simulink model "PracticaPotencia"  (R2024b)
settings: Solver=VariableStepAuto  StartTime=0.0  StopTime=200e-3  MaxStep=1e-4  RelTol=1e-3
libraries: spsVoltageMeasurementLib x14, spsDiodeLib x12, spsCurrentMeasurementLib x8, spsParallelRLCBranchLib x5, spsThreePhaseProgrammableVoltageSourceLib x2, spsMeanLib x1, spsRMSLib x1, sps_lib x1, spspowerguiLib x1
settings Model: Creator=javier  LastModifiedBy=javier

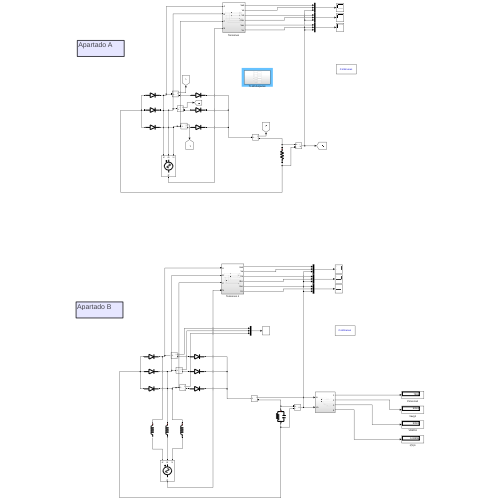
[thumbnail: Simulink's stored preview of the top-level diagram]
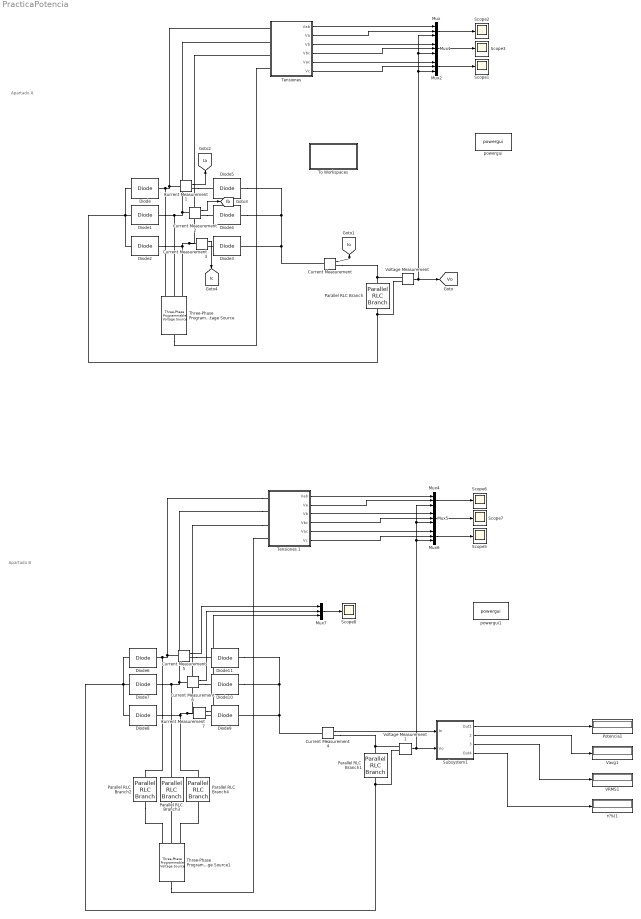
== system PracticaPotencia ==
  note: Apartado A
  note: Apartado B
  Current Measurement{,1..7} (8 alike) : spsCurrentMeasurementLib/Current Measurement  PhasorSimulation=off  OutputType=Complex  PSBequivalent=0
  Diode{,1..11} (12 alike) : spsDiodeLib/Diode  Ron=0.001  Lon=0  Vf=0.8  IC=0  UseSnubber=0  Rs=500  Cs=250e-9  Measurements=off
  Mux{,1..2,4..7} (7 alike) : Mux  Inputs=3
  Parallel RLC Branch : spsParallelRLCBranchLib/Parallel RLC Branch  LConnTagsString=a  RConnTagsString=__new0  BranchType=R  Resistance=30  Inductance=1e-3  SetiL0=off  InitialCurrent=0  Capacitance=1e-6  Setx0=off  InitialVoltage=0  Measurements=None
  Parallel RLC Branch1 : spsParallelRLCBranchLib/Parallel RLC Branch  LConnTagsString=a  RConnTagsString=__new0  BranchType=RC  Resistance=30  Inductance=1e-3  SetiL0=off  InitialCurrent=0  Capacitance=10e-3  Setx0=off  InitialVoltage=0  Measurements=None
  Parallel RLC Branch2 : spsParallelRLCBranchLib/Parallel RLC Branch  LConnTagsString=a  RConnTagsString=__new0  BranchType=L  Resistance=30  Inductance=5e-3  SetiL0=off  InitialCurrent=0  Capacitance=1e-6  Setx0=off  InitialVoltage=0  Measurements=None
  Parallel RLC Branch3 : spsParallelRLCBranchLib/Parallel RLC Branch  LConnTagsString=a  RConnTagsString=__new0  BranchType=L  Resistance=30  Inductance=5e-3  SetiL0=off  InitialCurrent=0  Capacitance=1e-6  Setx0=off  InitialVoltage=0  Measurements=None
  Parallel RLC Branch4 : spsParallelRLCBranchLib/Parallel RLC Branch  LConnTagsString=a  RConnTagsString=__new0  BranchType=L  Resistance=30  Inductance=5e-3  SetiL0=off  InitialCurrent=0  Capacitance=1e-6  Setx0=off  InitialVoltage=0  Measurements=None
  Potencia1 : Display
  Scope{1..3,5..8} (7 alike) : Scope
  Subsystem1 : Subsystem
  "Tensiones " : Subsystem
  Tensiones 1 : Subsystem
  Three-Phase Programmable Voltage Source : spsThreePhaseProgrammableVoltageSourceLib/Three-Phase Programmable Voltage Source  PositiveSequence="[400  0 50]"  VariationEntity=None  VariationType=Table of time-amplitude pairs  VariationTypeAlt=Step  VariationStep=0.5  VariationRate=10  VariationMagnitude=0.3  VariationFrequency=2  VariationTiming=[1 2]  VariationPhaseA=off  Amplitudes=[1 0.8 1.2 1.0]  TimeValues=[0 0.1 0.15 0.2]  HarmonicGeneration=off  HarmonicA=[3 0.2 -25 0]  HarmonicB=[2 0.15 35 2]  Timing="[0.05  3]"  BusType=swing  Pref=0  Qref=0  Qmin=-inf  Qmax=inf
  Three-Phase Programmable Voltage Source1 : spsThreePhaseProgrammableVoltageSourceLib/Three-Phase Programmable Voltage Source  PositiveSequence="[400  0 50]"  VariationEntity=None  VariationType=Table of time-amplitude pairs  VariationTypeAlt=Step  VariationStep=0.5  VariationRate=10  VariationMagnitude=0.3  VariationFrequency=2  VariationTiming=[1 2]  VariationPhaseA=off  Amplitudes=[1 0.8 1.2 1.0]  TimeValues=[0 0.1 0.15 0.2]  HarmonicGeneration=off  HarmonicA=[3 0.2 -25 0]  HarmonicB=[2 0.15 35 2]  Timing="[0.05  3]"  BusType=swing  Pref=0  Qref=0  Qmin=-inf  Qmax=inf
  To Workspaces : Subsystem
  VRMS1 : Display
  Vavg1 : Display
  Voltage Measurement : spsVoltageMeasurementLib/Voltage Measurement  PhasorSimulation=off  OutputType=Complex  PSBequivalent=0
  Voltage Measurement1 : spsVoltageMeasurementLib/Voltage Measurement  PhasorSimulation=off  OutputType=Complex  PSBequivalent=0
  powergui : sps_lib/powergui  Priority=1  SimulationMode=Continuous  SampleTime=50e-6  frequency=60  Iterations=50  frequencyindice=50  Pbase=100e6  ErrMax=1e-4  UnitsV=kV  UnitsW=MW  buscounter=0  FunctionMessages=off  echomessages=off  EnableUseOfTLC=off  CurrentSourceSwitches=off  DisableSnubberDevices=on  DisableRonSwitches=off  DisableVfSwitches=off  DisplayEquations=off  AutomaticDiscreteSolvers=off  SolverType=Tustin/Backward Euler (TBE)  Interpol=off  ExternalGateDelay=off  methode=off  Ts=100  x0status=blocks  SPID=on  SwTol=0  HookPort=off  NonlinearTolerance=1e-4  nMaxIteration=100  ContinueOnMaxIteration=off  RestoreLinks=warning  ResistiveCurrentMeasurement=off  Frange=[0:2:500]  Ylog=off  Xlog=on  ShowGrid=off  save=off  variable=ZData  structure=0  ZoomFFT=off  StartTime=0.0  cycles=1  DisplayStyle=1  fundamental=60  FreqAxis=off  MaxFrequency=1000  frequencyindicesteady=1  RmsSteady=1  display=off
  powergui1 : spspowerguiLib/powergui  Priority=1  SimulationMode=Continuous  SampleTime=50e-6  frequency=60  Iterations=50  frequencyindice=50  Pbase=100e6  ErrMax=1e-4  UnitsV=kV  UnitsW=MW  buscounter=0  FunctionMessages=off  echomessages=off  EnableUseOfTLC=off  CurrentSourceSwitches=off  DisableSnubberDevices=on  DisableRonSwitches=off  DisableVfSwitches=off  DisplayEquations=off  AutomaticDiscreteSolvers=off  SolverType=Tustin/Backward Euler (TBE)  Interpol=off  ExternalGateDelay=off  methode=off  Ts=100  x0status=blocks  SPID=on  SwTol=0  HookPort=off  NonlinearTolerance=1e-4  nMaxIteration=100  ContinueOnMaxIteration=off  RestoreLinks=warning  ResistiveCurrentMeasurement=off  Frange=[0:2:500]  Ylog=off  Xlog=on  ShowGrid=off  save=off  variable=ZData  structure=0  ZoomFFT=off  StartTime=0.0  cycles=1  DisplayStyle=1  fundamental=60  FreqAxis=off  MaxFrequency=1000  frequencyindicesteady=1  RmsSteady=1  display=off
  r(%)1 : Display
  tag scope: Ia=global, Ib=global, Ic=global, Io=global, Vo=global
  wires:
  Voltage Measurement/1 -> [Vo], Mux1/3, Mux/3, Mux2/3
  "Tensiones "/1(Vab) -> Mux/1
  "Tensiones "/2(Va) -> Mux/2
  "Tensiones "/3(Vb) -> Mux1/1
  "Tensiones "/4(Vbc) -> Mux1/2
  "Tensiones "/5(Vac) -> Mux2/1
  "Tensiones "/6(Vc) -> Mux2/2
  Mux/1 -> Scope2/1
  Mux1/1 -> Scope3/1
  Mux2/1 -> Scope1/1
  Current Measurement1/1 -> [Ia]
  Tensiones 1/1(Vab) -> Mux4/1
  Tensiones 1/6(Vc) -> Mux6/2
  Current Measurement4/1 -> Subsystem1/1(Io)
  Tensiones 1/3(Vb) -> Mux5/1
  Mux7/1 -> Scope8/1
  Tensiones 1/5(Vac) -> Mux6/1
  Current Measurement5/1 -> Mux7/1
  Subsystem1/2(2) -> Vavg1/1
  Mux5/1 -> Scope7/1
  Voltage Measurement1/1 -> Subsystem1/2(Vo), Mux5/3, Mux4/3, Mux6/3
  Mux6/1 -> Scope5/1
  Subsystem1/1(Out1) -> Potencia1/1
  Subsystem1/4(Out4) -> r(%)1/1
  Subsystem1/3(3) -> VRMS1/1
  Mux4/1 -> Scope6/1
  Current Measurement6/1 -> Mux7/2
  Current Measurement7/1 -> Mux7/3
  Tensiones 1/4(Vbc) -> Mux5/2
  Tensiones 1/2(Va) -> Mux4/2
  Current Measurement/1 -> [Io]
  Current Measurement2/1 -> [Ib]
  Current Measurement3/1 -> [Ic]
  connections:
  Voltage Measurement/LConn2 -- Parallel RLC Branch/RConn1 -- Diode2/LConn1 -- Diode1/LConn1 -- Diode/LConn1
  Diode5/RConn1 -- Current Measurement/LConn1 -- Diode3/RConn1 -- Diode4/RConn1
  Current Measurement/RConn1 -- Voltage Measurement/LConn1 -- Parallel RLC Branch/LConn1
  Three-Phase Programmable Voltage Source/LConn1 -- "Tensiones "/LConn4
  Diode/RConn1 -- Current Measurement1/LConn1 -- "Tensiones "/LConn1 -- Three-Phase Programmable Voltage Source/RConn1
  Diode1/RConn1 -- Current Measurement2/LConn1 -- "Tensiones "/LConn2 -- Three-Phase Programmable Voltage Source/RConn2
  Diode2/RConn1 -- Current Measurement3/LConn1 -- "Tensiones "/LConn3 -- Three-Phase Programmable Voltage Source/RConn3
  Current Measurement1/RConn1 -- Diode5/LConn1
  Current Measurement2/RConn1 -- Diode4/LConn1
  Current Measurement3/RConn1 -- Diode3/LConn1
  Tensiones 1/LConn1 -- Diode6/RConn1 -- Parallel RLC Branch2/LConn1 -- Current Measurement5/LConn1
  Tensiones 1/LConn2 -- Parallel RLC Branch3/LConn1 -- Diode7/RConn1 -- Current Measurement6/LConn1
  Diode6/LConn1 -- Voltage Measurement1/LConn2 -- Parallel RLC Branch1/RConn1 -- Diode8/LConn1 -- Diode7/LConn1
  Tensiones 1/LConn3 -- Parallel RLC Branch4/LConn1 -- Diode8/RConn1 -- Current Measurement7/LConn1
  Diode10/RConn1 -- Diode11/RConn1 -- Current Measurement4/LConn1 -- Diode9/RConn1
  Parallel RLC Branch1/LConn1 -- Current Measurement4/RConn1 -- Voltage Measurement1/LConn1
  Current Measurement6/RConn1 -- Diode10/LConn1
  Current Measurement7/RConn1 -- Diode9/LConn1
  Three-Phase Programmable Voltage Source1/LConn1 -- Tensiones 1/LConn4
  Current Measurement5/RConn1 -- Diode11/LConn1
  Parallel RLC Branch2/RConn1 -- Three-Phase Programmable Voltage Source1/RConn1
  Three-Phase Programmable Voltage Source1/RConn2 -- Parallel RLC Branch3/RConn1
  Three-Phase Programmable Voltage Source1/RConn3 -- Parallel RLC Branch4/RConn1

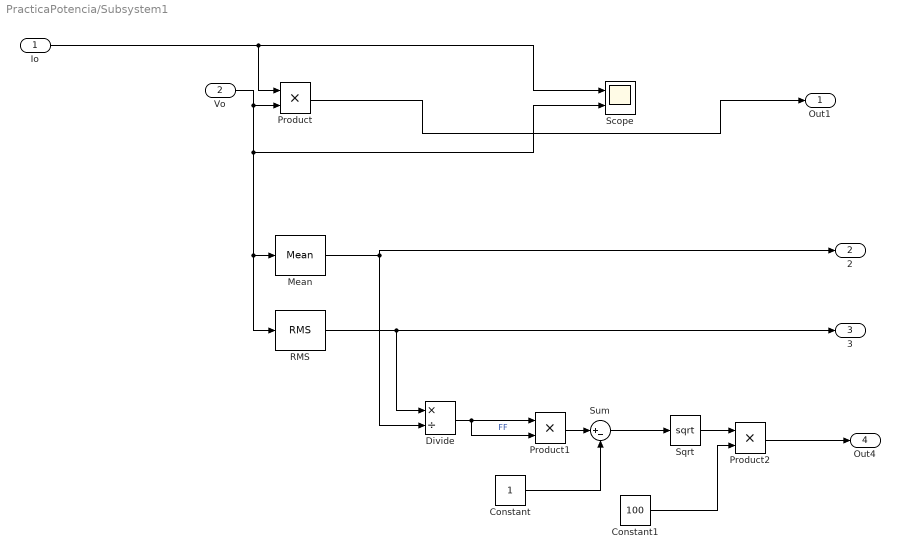
== system PracticaPotencia/Subsystem1 ==
  Io : Inport
  Vo : Inport  Port=2
  Constant : Constant
  Constant1 : Constant  Value=100
  Divide : Product  Inputs=*/
  Mean : spsMeanLib/Mean  Freq=50  Vinit=0  Ts=0
  Product : Product
  Product1 : Product
  Product2 : Product
  RMS : spsRMSLib/RMS  TrueRMS=on  Freq=50  RMSInit=120  Ts=0
  Scope : Scope  NumInputPorts=2
  Sqrt : Sqrt
  Sum : Sum  Inputs=|+-
  Out1 : Outport
  2 : Outport  Port=2
  3 : Outport  Port=3
  Out4 : Outport  Port=4
  wires:
  Vo/1 -> Scope/2, Mean/1, RMS/1, Product/2
  Constant/1 -> Sum/2
  Constant1/1 -> Product2/2
  RMS/1 -> 3/1, Divide/1
  Io/1 -> Scope/1, Product/1
  Divide/1 -> Product1/2, Product1/1  "FF"
  Sqrt/1 -> Product2/1
  Sum/1 -> Sqrt/1
  Mean/1 -> 2/1, Divide/2
  Product1/1 -> Sum/1
  Product/1 -> Out1/1
  Product2/1 -> Out4/1

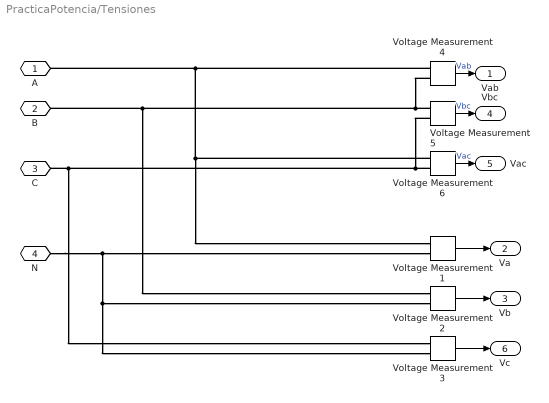
== system PracticaPotencia/Tensiones  ==
  Voltage Measurement{1..6} (6 alike) : spsVoltageMeasurementLib/Voltage Measurement  PhasorSimulation=off  OutputType=Complex  PSBequivalent=0
  A : PMIOPort  Side=Left
  B : PMIOPort  Port=2  Side=Left
  C : PMIOPort  Port=3  Side=Left
  N : PMIOPort  Port=4  Side=Left
  Vab : Outport
  Va : Outport  Port=2
  Vb : Outport  Port=3
  Vbc : Outport  Port=4
  Vac : Outport  Port=5
  Vc : Outport  Port=6
  wires:
  Voltage Measurement6/1 -> Vac/1  "Vac"
  Voltage Measurement5/1 -> Vbc/1  "Vbc"
  Voltage Measurement4/1 -> Vab/1  "Vab"
  Voltage Measurement1/1 -> Va/1
  Voltage Measurement2/1 -> Vb/1
  Voltage Measurement3/1 -> Vc/1
  connections:
  Voltage Measurement5/LConn2 -- Voltage Measurement6/LConn2 -- Voltage Measurement3/LConn1 -- C/RConn1
  Voltage Measurement4/LConn1 -- Voltage Measurement6/LConn1 -- Voltage Measurement1/LConn1 -- A/RConn1
  Voltage Measurement5/LConn1 -- Voltage Measurement4/LConn2 -- Voltage Measurement2/LConn1 -- B/RConn1
  N/RConn1 -- Voltage Measurement3/LConn2 -- Voltage Measurement2/LConn2 -- Voltage Measurement1/LConn2

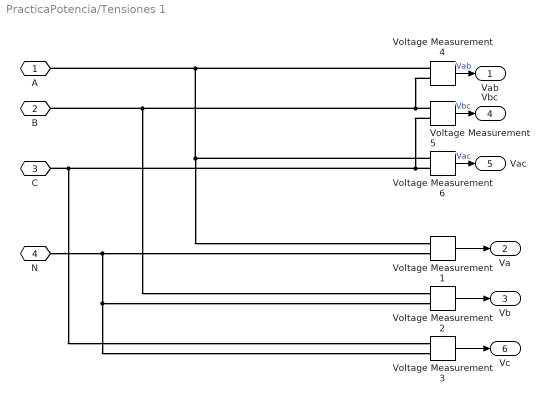
== system PracticaPotencia/Tensiones 1 ==
  Voltage Measurement{1..6} (6 alike) : spsVoltageMeasurementLib/Voltage Measurement  PhasorSimulation=off  OutputType=Complex  PSBequivalent=0
  A : PMIOPort  Side=Left
  B : PMIOPort  Port=2  Side=Left
  C : PMIOPort  Port=3  Side=Left
  N : PMIOPort  Port=4  Side=Left
  Vab : Outport
  Va : Outport  Port=2
  Vb : Outport  Port=3
  Vbc : Outport  Port=4
  Vac : Outport  Port=5
  Vc : Outport  Port=6
  wires:
  Voltage Measurement6/1 -> Vac/1  "Vac"
  Voltage Measurement5/1 -> Vbc/1  "Vbc"
  Voltage Measurement4/1 -> Vab/1  "Vab"
  Voltage Measurement1/1 -> Va/1
  Voltage Measurement2/1 -> Vb/1
  Voltage Measurement3/1 -> Vc/1
  connections:
  Voltage Measurement5/LConn2 -- Voltage Measurement6/LConn2 -- Voltage Measurement3/LConn1 -- C/RConn1
  Voltage Measurement4/LConn1 -- Voltage Measurement6/LConn1 -- Voltage Measurement1/LConn1 -- A/RConn1
  Voltage Measurement5/LConn1 -- Voltage Measurement4/LConn2 -- Voltage Measurement2/LConn1 -- B/RConn1
  N/RConn1 -- Voltage Measurement3/LConn2 -- Voltage Measurement2/LConn2 -- Voltage Measurement1/LConn2

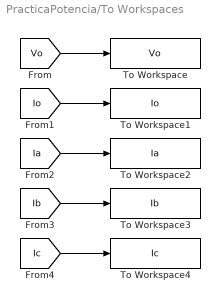
== system PracticaPotencia/To Workspaces ==
  To Workspace : ToWorkspace  VariableName=Vo  SampleTime=-1
  To Workspace1 : ToWorkspace  VariableName=Io  SampleTime=-1
  To Workspace2 : ToWorkspace  VariableName=Ia  SampleTime=-1
  To Workspace3 : ToWorkspace  VariableName=Ib  SampleTime=-1
  To Workspace4 : ToWorkspace  VariableName=Ic  SampleTime=-1
  wires:
  [Ic] -> To Workspace4/1
  [Vo] -> To Workspace/1
  [Ia] -> To Workspace2/1
  [Ib] -> To Workspace3/1
  [Io] -> To Workspace1/1
